simulink model "f18_SimulationModel"  (R2024a)
settings: Solver=ode1  StartTime=0.0  StopTime=200  FixedStep=0.01  RelTol=1e-3
values from neighbouring files (symbols this model uses):
  ALPHA_BREAK = [-14.0000  -10.00000   -6.00000   -2.00000    2.00000    6.00000     10.00000    14.0000    18.0000    22.0000    26.0000    30.0000    34.0000      38.0000    42.0000    46.0000    50.0000    54.0000    58.0000    62.0000      66.0000    70.0000    74.0000    78.0000    82.0000    86.0000    90.0000]*pi/180'    [f18_Aerodata.m]
  b = 37.4*0.3048    (= 11.39952)    [a1_initialize.m]
  cbar = 11.52*0.3048    (= 3.511296)    [a1_initialize.m]
  cd0 = [0.227325   0.170673    7.47685E-02    3.20977E-02    2.79305E-02  	     6.13288E-02   0.154023   0.261263   0.363863   0.486635   0.643989   0.863792  	     1.08558    1.27900    1.47638    1.61911    1.74604    1.84448    1.92402  	     1.98384    2.02834    2.06708    2.11362    2.15514    2.17363    2.16283  	     2.12822]    [f18_Aerodata.m]
  cd_de = cd_del+cd_der    [f18_Aerodata.m]
  cd_q = [ 1.48740E-16   -2.21604E-16   -8.70391E-05   -7.79330E-04   -8.31959E-04  	    -6.60720E-05    1.33279E-03    1.67685E-04    5.84481E-06   -9.59697E-17  	    -6.48262E-17   -2.05428E-16   -2.53047E-16    2.02363E-16    3.51664E-16  	     8.52635E-16    5.44982E-16   -5.45460E-16    1.14528E-15   -2.50755E-16  	     8.43503E-16   -8.45493E-16   -2.54842E-15   -7.66583E-16   -3.79368E-16  	     9.1 ...(+24 chars)    [f18_Aerodata.m]
  clift = [-1.03860  -0.880907  -0.551318  -0.216206   0.154461   0.560857  	     0.951575    1.24168    1.39786    1.53103    1.64110    1.77724    1.88652  	     1.88940    1.80975    1.68556    1.57524    1.46011    1.31884    1.17117  	     1.02151   0.858875   0.685334   0.529482   0.378268   0.229349    9.10933E-02]    [f18_Aerodata.m]
  clift_de = clift_del+clift_der    [f18_Aerodata.m]
  clift_q = [7.87143E-02    7.87143E-02    7.87144E-02    7.88452E-02    7.64891E-02  	     6.91587E-02    6.33554E-02    5.99084E-02    5.89049E-02    6.05629E-02  	     6.28755E-02    6.91587E-02    8.89245E-02    0.119991   0.147829   0.159698  	     0.131772       1.03847E-01    9.21534E-02    8.79646E-02    8.63938E-02    8.63938E-02  	     8.49975E-02    8.25541E-02    7.97615E-02    7.66200E-02    7.24 ...(+8 chars)    [f18_Aerodata.m]
  cm0 = [9.62520E-02    8.07290E-02    5.54066E-02    2.80686E-02    5.08503E-03  	    -6.61034E-03   -1.64371E-02   -1.60245E-02   -5.86329E-02   -8.42348E-02  	    -8.52663E-02  -0.105573  -0.117061  -0.110115  -0.114069  -0.118398   -1.01818E-01  	   -0.146057  -0.228343  -0.351592  -0.426319  -0.476887  -0.601749  -0.563499  	   -0.547688  -0.570013  -0.588038]    [f18_Aerodata.m]
  cm_de = cm_del+cm_der    [f18_Aerodata.m]
  cm_q = [-8.68301E-02   -8.68301E-02   -8.68301E-02   -8.65683E-02   -8.53902E-02  	    -8.08524E-02   -7.57473E-02   -7.23875E-02   -7.56600E-02   -8.29032E-02  	    -8.81828E-02   -1.02364E-01  -0.147655  -0.205556  -0.132732    1.80642E-02  	     4.31969E-02    1.80642E-02   -1.96350E-02   -6.50135E-02   -1.00967E-01  	    -9.81748E-02   -9.53822E-02   -9.25897E-02   -8.90991E-02   -8.52593E-02  	    - ...(+12 chars)    [f18_Aerodata.m]
  cn_b = [1.42071E-03    1.42071E-03    1.52521E-03    1.62971E-03    1.65089E-03  	    1.67084E-03    1.80024E-03    1.46016E-03    9.91781E-04    6.82316E-04  	    1.75902E-04   -1.09086E-03   -1.11070E-03   -1.59428E-03   -1.88776E-03  	   -1.76721E-03   -1.35917E-03   -1.52852E-03   -1.63273E-03   -1.59147E-03  	   -1.44456E-03   -1.34440E-03   -1.47796E-03   -1.60891E-03   -1.69618E-03  	    -1.72843E ...(+19 chars)    [f18_Aerodata.m]
  cn_da = [-8.69999E-06   -8.69999E-06   -8.69999E-06   -2.06625E-05   -3.45825E-05  	    -3.93675E-05   -4.78500E-05   -6.15525E-05   -7.74300E-05   -1.02660E-04  	    -1.32240E-04   -1.55512E-04   -1.72042E-04   -1.80090E-04   -1.97403E-04  	    -2.05320E-04   -2.40120E-04   -2.69352E-04   -2.87796E-04   -3.02644E-04  	    -1.09272E-04    2.45624E-12    8.35200E-05    1.59210E-04    2.21850E-04  	     2.4 ...(+24 chars)    [f18_Aerodata.m]
  cn_de = cn_del+cn_der    [f18_Aerodata.m]
  cn_dr = [-1.15493E-03   -1.15493E-03   -1.15493E-03   -1.16632E-03   -1.18177E-03  	    -1.18259E-03   -1.15656E-03   -1.08336E-03   -9.58920E-04   -8.03573E-04  	    -6.80760E-04   -6.18947E-04   -5.90480E-04   -5.80720E-04   -5.15533E-04  	    -4.17092E-04   -3.72355E-04   -3.86914E-04   -3.85538E-04   -3.51603E-04  	    -3.00387E-04   -2.75612E-04   -2.70873E-04   -3.22200E-04   -3.84710E-04  	    -4.2 ...(+24 chars)    [f18_Aerodata.m]
  cn_p = [-1.26406E-03   -1.26406E-03   -1.26406E-03   -1.23533E-03   -1.17787E-03  	    -1.12041E-03   -9.39611E-04   -6.36739E-04   -2.47236E-04    1.00356E-04  	     3.70882E-04    4.58149E-04    3.97062E-04    2.48709E-04    2.33874E-04  	     4.18879E-04    6.98132E-04    9.77384E-04   -1.04720E-03   -1.60570E-03  	    -3.24631E-04   -2.26893E-04   -1.44164E-03   -6.98132E-04   -8.81388E-14  	    -9.3 ...(+24 chars)    [f18_Aerodata.m]
  cn_r = [-3.11978E-03   -3.11978E-03   -3.11978E-03   -3.11105E-03   -3.10669E-03  	    -3.12850E-03   -3.17650E-03   -3.27686E-03   -3.46448E-03   -3.97935E-03  	    -4.62949E-03   -5.14872E-03   -5.53269E-03   -5.63741E-03   -5.53706E-03  	    -5.23162E-03   -4.53349E-03   -3.97499E-03   -2.89288E-03   -1.70606E-03  	    -6.93768E-04    4.36324E-06   -6.93769E-04   -2.64854E-03   -4.18443E-03  	    -4.8 ...(+24 chars)    [f18_Aerodata.m]
  croll_b = [-3.70196E-05   -3.70196E-05   -4.41520E-04   -8.46019E-04   -1.27065E-03  	   -1.70123E-03   -2.11290E-03   -2.77077E-03   -3.37291E-03   -3.47757E-03  	   -3.16486E-03   -2.35754E-03   -1.22554E-03   -1.14567E-03   -1.63756E-03  	   -2.22957E-03   -2.45882E-03   -2.47686E-03   -2.44493E-03   -2.51646E-03  	   -2.70976E-03   -2.90803E-03   -2.82658E-03   -2.75756E-03   -2.70552E-03  	   -2.67292E ...(+19 chars)    [f18_Aerodata.m]
  croll_da = [1.16543E-03    1.16543E-03    1.16543E-03    1.16686E-03    1.17021E-03  	    1.17426E-03    1.14013E-03    1.04034E-03    8.40294E-04    6.31892E-04  	    5.23513E-04    4.56671E-04    3.86010E-04    3.20124E-04    2.81594E-04  	    2.56481E-04    2.33946E-04    2.11792E-04    1.97660E-04    1.86966E-04  	    1.74839E-04    1.56123E-04    9.61564E-05    5.02267E-05    1.77607E-05  	   -6.65660E- ...(+18 chars)    [f18_Aerodata.m]
  croll_de = croll_del+croll_der    [f18_Aerodata.m]
  croll_dr = [2.86293E-04    2.86293E-04    2.86293E-04    2.69213E-04    2.39120E-04  	    2.18787E-04    2.10653E-04    2.07400E-04    1.80560E-04    1.24440E-04  	    6.91333E-05    3.49733E-05    1.87067E-05    4.88000E-06   -3.44528E-05  	   -8.67339E-05   -1.08661E-04   -7.83403E-05   -2.63520E-05    3.68277E-05  	    9.48021E-05    1.25253E-04    9.58432E-05    7.66811E-05    6.73115E-05  	    6.47088E- ...(+18 chars)    [f18_Aerodata.m]
  croll_p = [-7.05113E-03   -7.05113E-03   -7.05113E-03   -7.05113E-03   -7.05113E-03  	   -7.05113E-03   -6.24828E-03   -5.25344E-03   -4.62512E-03   -3.85718E-03  	   -5.38434E-03   -7.94125E-03   -8.68301E-03   -8.72665E-03   -4.88692E-03  	    3.49064E-05   -3.31613E-03   -3.73500E-03   -4.04916E-03   -4.36332E-03  	   -4.67748E-03   -4.88692E-03   -5.02655E-03   -5.16617E-03   -5.30580E-03  	   -5.41052E ...(+19 chars)    [f18_Aerodata.m]
  croll_r = [2.14676E-04    2.14676E-04    2.14676E-04    5.85558E-04    1.52804E-03  	    2.57087E-03    3.39117E-03    3.84496E-03    3.98895E-03    4.11549E-03  	    4.43401E-03    5.18886E-03    5.68192E-03    5.06669E-03    4.07360E-03  	    3.28122E-03    2.56214E-03    2.18515E-03    1.86052E-03    1.58127E-03  	    1.33692E-03    1.11352E-03    1.12748E-03    1.13097E-03    9.28515E-04  	    5.34071E- ...(+18 chars)    [f18_Aerodata.m]
  cy_b = [-1.71957E-02   -1.71957E-02   -1.77407E-02   -1.82857E-02   -1.84197E-02  	   -1.84159E-02   -1.87763E-02   -1.77142E-02   -1.55057E-02   -1.40980E-02  	   -1.28732E-02   -1.26852E-02   -1.25160E-02   -1.35594E-02   -1.40314E-02  	   -1.33128E-02   -1.19496E-02   -1.30678E-02   -1.37112E-02   -1.37528E-02  	   -1.33426E-02   -1.29076E-02   -1.33076E-02   -1.38320E-02   -1.37811E-02  	   -1.31714E ...(+19 chars)    [f18_Aerodata.m]
  cy_da = [-5.77397E-04   -5.77397E-04   -5.77397E-04   -5.46240E-04   -4.60488E-04  	   -4.06750E-04   -4.16183E-04   -3.70449E-04   -1.95515E-04    4.51627E-05  	    2.63830E-04    4.73923E-04    6.38852E-04    7.09741E-04    6.50343E-04  	    1.99345E-04   -1.00616E-04   -1.48179E-04   -1.74477E-04   -1.95743E-04  	   -2.18725E-04   -2.40677E-04   -2.78179E-04   -3.06420E-04   -3.28602E-04  	   -3.47581E ...(+19 chars)    [f18_Aerodata.m]
  cy_de = cy_del+cy_der    [f18_Aerodata.m]
  cy_dr = [3.46480E-03    3.46480E-03    3.46480E-03    3.52987E-03    3.66813E-03  	    3.73320E-03    3.66813E-03    3.46480E-03    3.08253E-03    2.57827E-03  	    2.11467E-03    1.79747E-03    1.59413E-03    1.47213E-03    1.50955E-03  	    1.59771E-03    1.48189E-03    1.25806E-03    1.04497E-03    9.72747E-04  	    1.04790E-03    1.15331E-03    1.10125E-03    1.01504E-03    1.04757E-03  	    1.15266E- ...(+18 chars)    [f18_Aerodata.m]
  cy_p = [-1.06465E-03   -1.06465E-03   -1.06465E-03   -8.63938E-04   -2.09440E-04  	    4.14516E-04    5.80322E-04    5.32325E-04    4.53786E-04    2.22529E-04  	   -1.74533E-04   -5.49779E-04   -9.42478E-04   -1.35699E-03   -2.60752E-03  	   -4.39823E-03   -5.23599E-03   -3.00197E-03   -1.65806E-03   -7.85399E-04  	   -2.96706E-04   -4.36332E-04   -9.25024E-04   -9.94838E-04   -9.25024E-04  	   -9.77384E ...(+19 chars)    [f18_Aerodata.m]
  cy_r = [2.69653E-03    2.69653E-03    2.69653E-03    2.89725E-03    3.36412E-03  	    3.94444E-03    4.45932E-03    3.82227E-03    1.22609E-03   -1.61443E-03  	   -3.46448E-03   -4.66876E-03   -5.36689E-03   -5.67232E-03   -3.89208E-03  	    3.49069E-05    5.06146E-03    5.06145E-03    4.11898E-03    2.79253E-03  	    1.60570E-03    1.04720E-03    8.37758E-04    6.28319E-04    4.88692E-04  	    4.18879E- ...(+18 chars)    [f18_Aerodata.m]
  g = 9.80665    [a1_initialize.m]
  InertiaTensor = [Ixx 0 -Ixz; 0 Iyy 0; -Ixz 0 Izz]    [a1_initialize.m]
  init_eulers = x0(7:9)    [a1_initialize.m]
  init_inertial = x0(10:12)    [a1_initialize.m]
  init_omega_b = x0(1:3)    [a1_initialize.m]
  init_Vb = x0(4:6)    [a1_initialize.m]
  mass = 36100/2.2046    (= 16374.852581)    [a1_initialize.m]
  max_thrust = 32000*g/2.2046    (= 142344.5523)    [a1_initialize.m]
  rho_sl = 1.225    [a1_initialize.m]
  S = 400.0*0.3048*0.3048    (= 37.161216)    [a1_initialize.m]
undefined symbols (not defined in the file or in its folder): Earth, WGS84
libraries: aerolibfltsims x2, matrix_library x2, aerolibtransform2 x1, Rotation_Matrices_All x1
(part 1 of 2)
settings Model: Creator=ragup  LastModifiedBy=ragup
settings DataIOCC: ExternalInput=getinputstruct(opreport)  InitialState=getstatestruct(opreport)  LoadExternalInput=on  LoadInitialState=on  SaveOutput=off  SignalLogging=off  DSMLogging=off  SaveTime=off  ReturnWorkspaceOutputs=off

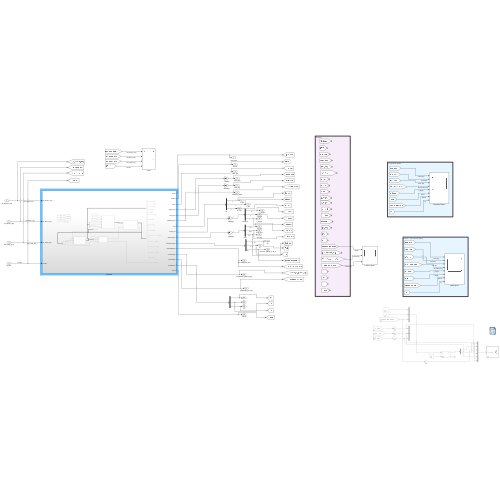
[thumbnail: Simulink's stored preview of the top-level diagram]
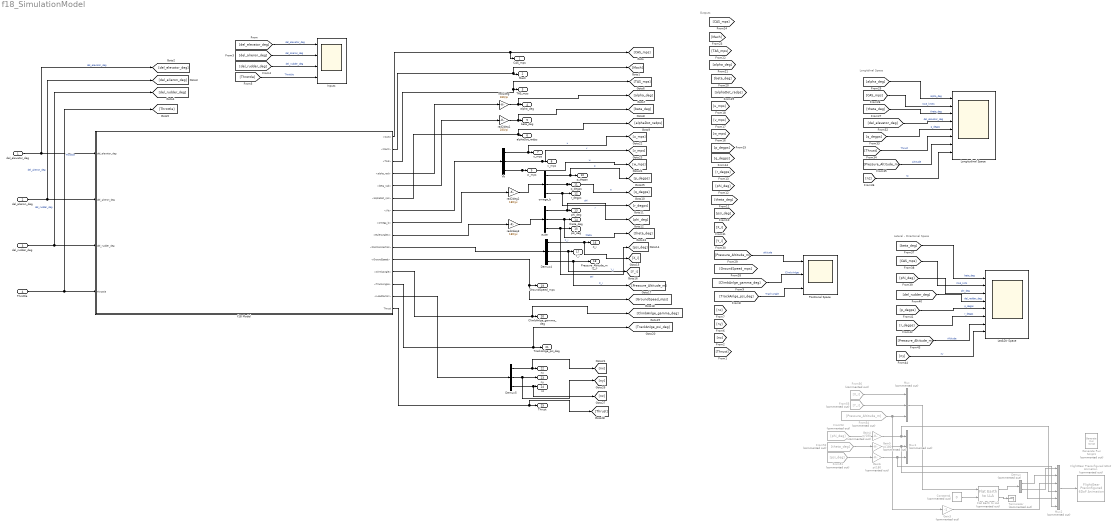
== system f18_SimulationModel ==
  note: Outputs
  note: Longitdinal Space
  note: Lateral - Directional Space
  del_elevator_deg : Inport
  del_alieron_deg : Inport  Port=2
  del_rudder_deg : Inport  Port=3
  Throttle : Inport  Port=4
  Constant4 : Constant  Commented=on  Value=0
  Demux : Demux  Commented=on  Outputs=2
  Demux4 : Demux  Outputs=3
  Demux5 : Demux  Outputs=3
  Flat Earth to LLA : aerolibtransform2/Flat Earth to LLA  Commented=on  units=Metric (MKS)  ptype=Earth (WGS84)  F=1/298.257223563  R=6378137  refPosPort=off  LL0=[63 -22]  psi=0
  FlightGear Preconfigured 6DoF Animation : aerolibfltsims/FlightGear Preconfigured 6DoF Animation  Commented=on  xFlightGearVersion=v2019.1  DestinationIpAddress=127.0.0.1  DestinationPort=5502  SampleTime=0.01  packetVersion=24
  From51 : From  Commented=on  GotoTag=psi_deg
  From52 : From  Commented=on  GotoTag=theta_deg
  From53 : From  Commented=on  GotoTag=phi_deg
  From54 : From  Commented=on  GotoTag=Pressure_Altitude_m
  From55 : From  Commented=on  GotoTag=Y_i
  From56 : From  Commented=on  GotoTag=X_i
  Gain3 : Gain  Commented=on  Gain=-1
  Gain4 : Gain  Commented=on  Gain=pi/180
  Gain5 : Gain  Commented=on  Gain=pi/180
  Gain6 : Gain  Commented=on  Gain=pi/180
  Generate Run Script1 : aerolibfltsims/Generate Run Script  Commented=on  Architecture=Win64  dataFlow=Send  GeometryModelName=c172p  AirportId=BIKF  RunwayId=10  InitialAltitude=2000  InitialHeading=0  OffsetDistance=4.7  OffsetAzimuth=0  InstallScenery=off  DisableShaders=off  OriginAddress=127.0.0.1  DestinationPort=5502  OriginPort=5505  LocalAddress=127.0.0.1  OutputFileName=runfg_f18.bat  FlightGearBaseDirectory=C:\Program Files\FlightGear
  Inputs : Scope  NumInputPorts=4
  Lat&Dir Space : Scope  NumInputPorts=8
  Longitudinal Space : Scope  NumInputPorts=8
  Mux : Mux  Commented=on  Inputs=3
  Mux1 : Mux  Commented=on  Inputs=3
  Mux2 : Mux  Commented=on  Inputs=6
  Positional Space : Scope  NumInputPorts=3
  Terminator : Terminator  Commented=on
  Vb : Demux  Outputs=3
  euler : Demux  Outputs=3
  f18 Model : Subsystem
  omega_b : Demux  Outputs=3
  rad2deg{,1..3} (4 alike) : Gain  Gain=180/pi
  CAS_mps : Outport
  Mach : Outport  Port=2
  TAS_mps : Outport  Port=3
  alpha_deg : Outport  Port=4
  beta_deg : Outport  Port=5
  alphaDot_radps : Outport  Port=6
  u_mps : Outport  Port=7
  v_mps : Outport  Port=8
  w_mps : Outport  Port=9
  p_degps : Outport  Port=10
  q_degps : Outport  Port=11
  r_degps : Outport  Port=12
  phi_deg : Outport  Port=13
  theta_deg : Outport  Port=14
  psi_deg : Outport  Port=15
  X_i : Outport  Port=16
  Y_i : Outport  Port=17
  Pressure_Altitude_m (Z_i) : Outport  Port=18
  GroundSpeed_mps : Outport  Port=19
  ClimbAnlge_gamma_deg : Outport  Port=20
  TrackAnlge_psi_deg : Outport  Port=21
  nx : Outport  Port=22
  ny : Outport  Port=23
  nz : Outport  Port=24
  Thrust : Outport  Port=25
  wires:
  rad2deg/1 -> [alpha_deg], alpha_deg/1
  rad2deg1/1 -> [beta_deg], beta_deg/1
  Vb/1 -> [u_mps], u_mps/1  "u"
  Vb/2 -> [v_mps], v_mps/1  "v"
  Vb/3 -> [w_mps], w_mps/1  "w"
  omega_b/3 -> [r_degps], r_degps/1  "r"
  omega_b/2 -> [q_degps], q_degps/1  "q"
  omega_b/1 -> [p_degps], p_degps/1  "p"
  rad2deg2/1 -> omega_b/1
  rad2deg3/1 -> euler/1
  euler/1 -> [phi_deg], phi_deg/1  "phi"
  euler/2 -> [theta_deg], theta_deg/1  "theta"
  euler/3 -> [psi_deg], psi_deg/1  "psi"
  Demux4/3 -> Pressure_Altitude_m (Z_i)/1, [Pressure_Altitude_m]  "Z_i"
  Demux4/2 -> [Y_i], Y_i/1  "Y_i"
  Demux4/1 -> [X_i], X_i/1  "X_i"
  Demux5/3 -> [nz], nz/1
  Demux5/1 -> [nx], nx/1
  Demux5/2 -> ny/1, [ny]
  [beta_deg] -> Lat&Dir Space/1  "beta_deg"
  [q_degps] -> Longitudinal Space/5  "q_degps"
  [nz] -> Longitudinal Space/8  "nz"
  [Pressure_Altitude_m] -> Longitudinal Space/7  "Altitude"
  [theta_deg] -> Longitudinal Space/3  "theta_deg"
  [alpha_deg] -> Longitudinal Space/1  "alpha_deg"
  [del_rudder_deg] -> Lat&Dir Space/4  "del_redder_deg"
  [Pressure_Altitude_m] -> Lat&Dir Space/7  "Altitude"
  [ny] -> Lat&Dir Space/8  "ny"
  [r_degps] -> Lat&Dir Space/6  "r_degps"
  [CAS_mps] -> Lat&Dir Space/2  "CAS_knts"
  [CAS_mps] -> Longitudinal Space/2  "CAS_knots"
  [del_elevator_deg] -> Longitudinal Space/4  "del_elevator_deg"
  [p_degps] -> Lat&Dir Space/5  "p_degps"
  [Thrust] -> Longitudinal Space/6  "Thrust"
  [phi_deg] -> Lat&Dir Space/3  "phi_deg"
  f18 Model/15(Thrust) -> [Thrust], Thrust/1
  f18 Model/12(<ClimbAngle>) -> [ClimbAnlge_gamma_deg], ClimbAnlge_gamma_deg/1
  f18 Model/13(<TrackAngle>) -> [TrackAnlge_psi_deg], TrackAnlge_psi_deg/1
  f18 Model/11(<GroundSpeed>) -> GroundSpeed_mps/1, [GroundSpeed_mps]
  f18 Model/2(<Mach>) -> [Mach], Mach/1
  f18 Model/3(<TAS>) -> [TAS_mps], TAS_mps/1
  f18 Model/1(<CAS>) -> CAS_mps/1, [CAS_mps]
  f18 Model/6(<alphaDot_rps>) -> [alphaDot_radps], alphaDot_radps/1
  f18 Model/4(<alpha_rad>) -> rad2deg/1
  f18 Model/5(<beta_rad>) -> rad2deg1/1
  f18 Model/7(<Vb>) -> Vb/1
  f18 Model/8(<omega_b>) -> rad2deg2/1
  f18 Model/9(<EulerAngles>) -> rad2deg3/1
  f18 Model/10(<PositionInertial>) -> Demux4/1
  f18 Model/14(<LoadFactor>) -> Demux5/1
  Flat Earth to LLA/1 -> Demux/1
  Gain5/1 -> Mux2/5, Mux1/2
  Gain6/1 -> Mux1/3, Mux2/6
  Gain3/1 -> Mux2/3
  Gain4/1 -> Mux2/4, Mux1/1
  From56/1 -> Mux/1
  Mux2/1 -> FlightGear Preconfigured 6DoF Animation/1
  Flat Earth to LLA/2 -> Terminator/1
  Demux/2 -> Mux2/1
  From52/1 -> Gain5/1
  Constant4/1 -> Flat Earth to LLA/2
  Mux/1 -> Flat Earth to LLA/1
  From51/1 -> Gain6/1
  From53/1 -> Gain4/1
  Demux/1 -> Mux2/2
  From54/1 -> Gain3/1, Mux/3
  From55/1 -> Mux/2
  [del_elevator_deg] -> Inputs/1  "del_elevator_deg"
  [del_alieron_deg] -> Inputs/2  "del_alieron_deg"
  [del_rudder_deg] -> Inputs/3  "del_rudder_deg"
  [Throttle] -> Inputs/4  "Throttle"
  del_elevator_deg/1 -> [del_elevator_deg], f18 Model/1(del_elevator_deg)  "del_elevator_deg"
  del_alieron_deg/1 -> [del_alieron_deg], f18 Model/2(del_alieron_deg)  "del_alieron_deg"
  del_rudder_deg/1 -> [del_rudder_deg], f18 Model/3(del_rudder_deg)  "del_rudder_deg"
  Throttle/1 -> [Throttle], f18 Model/4(Throttle)  "Throttle"
  [ClimbAnlge_gamma_deg] -> Positional Space/2  "Climb Anlge"
  [TrackAnlge_psi_deg] -> Positional Space/3  "Trach Angle"
  [Pressure_Altitude_m] -> Positional Space/1  "altitude"

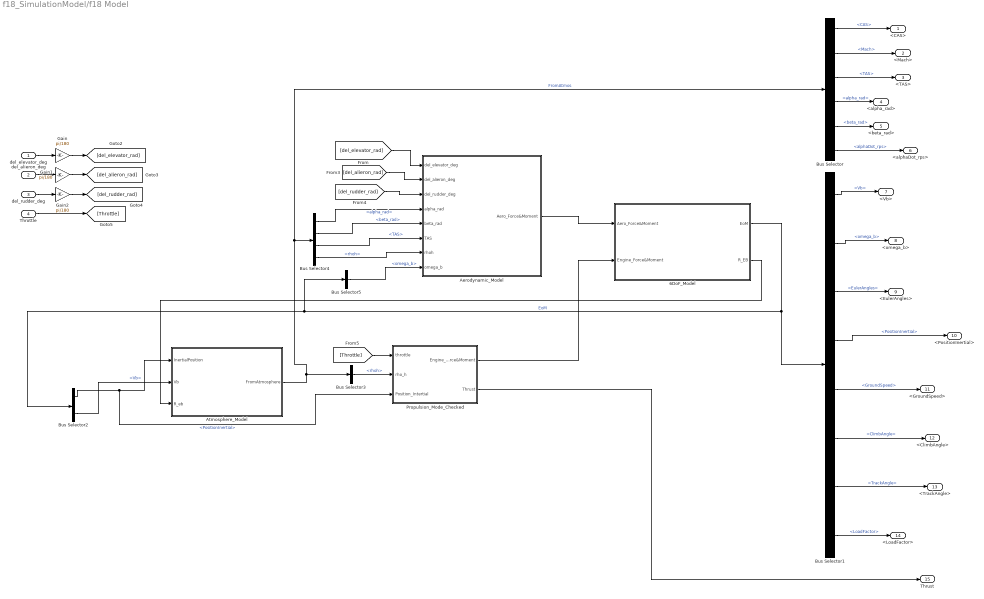
== system f18_SimulationModel/f18 Model ==
  del_elevator_deg : Inport
  del_alieron_deg : Inport  Port=2
  del_rudder_deg : Inport  Port=3
  Throttle : Inport  Port=4
  6DoF_Model : Subsystem
  Aerodynamic_Model : Subsystem
  Atmosphere_Model : Subsystem
  Bus Selector : BusSelector  OutputSignals=CAS,Mach,TAS,alpha_rad,beta_rad,alphaDot_rps
  Bus Selector1 : BusSelector  OutputSignals=Vb,omega_b,EulerAngles,PositionInertial,GroundSpeed,ClimbAngle,TrackAngle,LoadFactor
  Bus Selector2 : BusSelector  OutputSignals=PositionInertial,Vb
  Bus Selector3 : BusSelector  OutputSignals=rhoh
  Bus Selector4 : BusSelector  OutputSignals=alpha_rad,beta_rad,TAS,rhoh
  Bus Selector5 : BusSelector  OutputSignals=omega_b
  Gain : Gain  Gain=pi/180
  Gain1 : Gain  Gain=pi/180
  Gain2 : Gain  Gain=pi/180
  Propulsion_Mode_Checked : Subsystem
  <CAS> : Outport
  <Mach> : Outport  Port=2
  <TAS> : Outport  Port=3
  <alpha_rad> : Outport  Port=4
  <beta_rad> : Outport  Port=5
  <alphaDot_rps> : Outport  Port=6
  <Vb> : Outport  Port=7
  <omega_b> : Outport  Port=8
  <EulerAngles> : Outport  Port=9
  <PositionInertial> : Outport  Port=10
  <GroundSpeed> : Outport  Port=11
  <ClimbAngle> : Outport  Port=12
  <TrackAngle> : Outport  Port=13
  <LoadFactor> : Outport  Port=14
  Thrust : Outport  Port=15
  wires:
  Atmosphere_Model/1(FromAtmosphere) -> Bus Selector/1, Bus Selector4/1, Bus Selector3/1  "FromAtmos"
  Bus Selector4/1 -> Aerodynamic_Model/4(alpha_rad)  "<alpha_rad>"
  Propulsion_Mode_Checked/1(Engine_Force&Moment) -> 6DoF_Model/2(Engine_Force&Moment)
  Bus Selector2/2 -> Atmosphere_Model/2(Vb)  "<Vb>"
  Aerodynamic_Model/1(Aero_Force&Moment) -> 6DoF_Model/1(Aero_Force&Moment)
  Propulsion_Mode_Checked/2(Thrust) -> Thrust/1
  [del_elevator_rad] -> Aerodynamic_Model/1(del_elevator_deg)
  Bus Selector1/7 -> <TrackAngle>/1  "<TrackAngle>"
  del_elevator_deg/1 -> Gain/1
  Bus Selector/2 -> <Mach>/1  "<Mach>"
  [del_rudder_rad] -> Aerodynamic_Model/3(del_rudder_deg)
  Bus Selector/6 -> <alphaDot_rps>/1  "<alphaDot_rps>"
  Bus Selector3/1 -> Propulsion_Mode_Checked/2(rho_h)  "<rhoh>"
  del_alieron_deg/1 -> Gain1/1
  Bus Selector4/3 -> Aerodynamic_Model/6(TAS)  "<TAS>"
  Bus Selector4/4 -> Aerodynamic_Model/7(rhoh)  "<rhoh>"
  Bus Selector4/2 -> Aerodynamic_Model/5(beta_rad)  "<beta_rad>"
  Bus Selector2/1 -> Propulsion_Mode_Checked/3(Position_Intertial), Atmosphere_Model/1(InertialPosition)  "<PositionInertial>"
  6DoF_Model/1(EoM) -> Bus Selector5/1, Bus Selector2/1, Bus Selector1/1  "EoM"
  [del_alieron_rad] -> Aerodynamic_Model/2(del_alieron_deg)
  Bus Selector5/1 -> Aerodynamic_Model/8(omega_b)  "<omega_b>"
  Bus Selector1/8 -> <LoadFactor>/1  "<LoadFactor>"
  6DoF_Model/2(R_EB) -> Atmosphere_Model/3(R_eb)
  Bus Selector1/2 -> <omega_b>/1  "<omega_b>"
  [Throttle] -> Propulsion_Mode_Checked/1(throttle)
  del_rudder_deg/1 -> Gain2/1
  Bus Selector1/5 -> <GroundSpeed>/1  "<GroundSpeed>"
  Bus Selector/4 -> <alpha_rad>/1  "<alpha_rad>"
  Throttle/1 -> [Throttle]
  Bus Selector1/1 -> <Vb>/1  "<Vb>"
  Bus Selector1/3 -> <EulerAngles>/1  "<EulerAngles>"
  Bus Selector1/6 -> <ClimbAngle>/1  "<ClimbAngle>"
  Bus Selector1/4 -> <PositionInertial>/1  "<PositionInertial>"
  Bus Selector/1 -> <CAS>/1  "<CAS>"
  Bus Selector/3 -> <TAS>/1  "<TAS>"
  Bus Selector/5 -> <beta_rad>/1  "<beta_rad>"
  Gain/1 -> [del_elevator_rad]
  Gain1/1 -> [del_alieron_rad]
  Gain2/1 -> [del_rudder_rad]

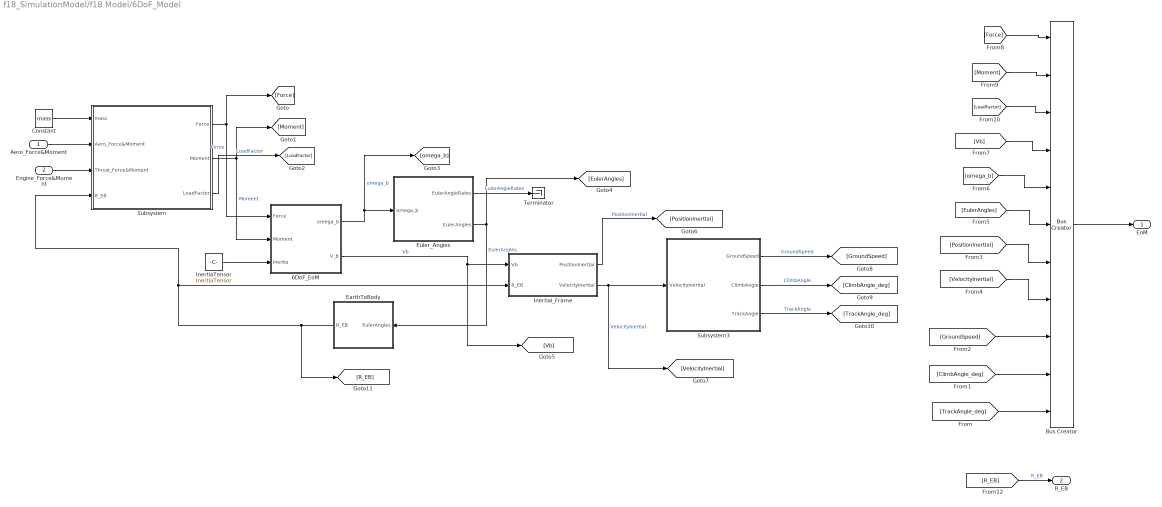
== system f18_SimulationModel/f18 Model/6DoF_Model ==
  Aero_Force&Moment : Inport
  Engine_Force&Moment : Inport  Port=2
  6DoF_EoM : Subsystem
  Bus Creator : BusCreator  Inputs=11
  Constant : Constant  Value=mass
  EarthToBody : Subsystem
  Euler_Angles : Subsystem
  InertiaTensor : Constant  Value=InertiaTensor  VectorParams1D=off
  Inertial_Frame : Subsystem
  Subsystem : Subsystem
  Subsystem3 : Subsystem
  Terminator : Terminator
  EoM : Outport
  R_EB : Outport  Port=2
  wires:
  [ClimbAngle_deg] -> Bus Creator/10
  [LoadFactor] -> Bus Creator/3
  [Moment] -> Bus Creator/2
  Bus Creator/1 -> EoM/1
  Subsystem/3(LoadFactor) -> [LoadFactor]  "LoadFactor"
  [PositionInertial] -> Bus Creator/7
  Inertial_Frame/1(PositionInertial) -> [PositionInertial]  "PositionInertial"
  [omega_b] -> Bus Creator/5
  EarthToBody/1(R_EB) -> [R_EB], Inertial_Frame/2(R_EB), Subsystem/4(R_EB)
  Euler_Angles/1(EulerAngleRates) -> Terminator/1  "EulerAngleRates"
  Subsystem3/1(GroundSpeed) -> [GroundSpeed]  "GroundSpeed"
  Aero_Force&Moment/1 -> Subsystem/2(Aero_Force&Moment)
  Subsystem3/2(ClimbAngle) -> [ClimbAngle_deg]  "ClimbAngle"
  [EulerAngles] -> Bus Creator/6
  [VelocityInertial] -> Bus Creator/8
  [GroundSpeed] -> Bus Creator/9
  6DoF_EoM/2(V_b) -> Inertial_Frame/1(Vb), [Vb]  "Vb"
  Engine_Force&Moment/1 -> Subsystem/3(Thrust_Force&Moment)
  [Force] -> Bus Creator/1
  Constant/1 -> Subsystem/1(mass)
  Inertial_Frame/2(VelocityInertial) -> Subsystem3/1(VelocityInertial), [VelocityInertial]  "VelocityInertial"
  [TrackAngle_deg] -> Bus Creator/11
  [Vb] -> Bus Creator/4
  6DoF_EoM/1(omega_b) -> [omega_b], Euler_Angles/1(omega_b)  "omega_b"
  Euler_Angles/2(EulerAngles) -> [EulerAngles], EarthToBody/1(EulerAngles)  "EulerAngles"
  Subsystem/2(Moment) -> [Moment], 6DoF_EoM/2(Moment)  "Moment"
  Subsystem3/3(TrackAngle) -> [TrackAngle_deg]  "TrackAngle"
  Subsystem/1(Force) -> [Force], 6DoF_EoM/1(Force)  "Force"
  [R_EB] -> R_EB/1  "R_EB"
  InertiaTensor/1 -> 6DoF_EoM/3(Inertia)

== system f18_SimulationModel/f18 Model/Aerodynamic_Model ==
  del_elevator_deg : Inport
  del_alieron_deg : Inport  Port=2
  del_rudder_deg : Inport  Port=3
  alpha_rad : Inport  Port=4
  beta_rad : Inport  Port=5
  TAS : Inport  Port=6
  rhoh : Inport  Port=7
  omega_b : Inport  Port=8
  Absolute Force&Moment : Subsystem
  Bus Creator1 : BusCreator  Inputs=6
  Co-efficent Calculation in body FoR : Subsystem
  Demux : Demux  Outputs=3
  Demux4 : Demux  Outputs=2
  Demux5 : Demux  Outputs=3
  Demux6 : Demux  Outputs=3
  Stability FoR to Body FoR : Subsystem
  Aero_Force&Moment : Outport
  wires:
  Demux/1 -> Co-efficent Calculation in body FoR/3(p)  "p"
  omega_b/1 -> Demux/1
  [TAS] -> Co-efficent Calculation in body FoR/9(TAS)
  TAS/1 -> [TAS]
  rhoh/1 -> [rhoh]
  Demux/2 -> Co-efficent Calculation in body FoR/4(q)  "q"
  alpha_rad/1 -> Stability FoR to Body FoR/1(alpha_rad), Co-efficent Calculation in body FoR/1(alpha_rad)
  del_alieron_deg/1 -> Co-efficent Calculation in body FoR/7(del_alieron_deg)
  Demux/3 -> Co-efficent Calculation in body FoR/5(r)  "r"
  del_elevator_deg/1 -> Co-efficent Calculation in body FoR/6(del_elevator_deg)
  beta_rad/1 -> Co-efficent Calculation in body FoR/2(beta_rad)
  del_rudder_deg/1 -> Co-efficent Calculation in body FoR/8(del_rudder_deg)
  Bus Creator1/1 -> Aero_Force&Moment/1
  Demux4/1 -> Demux5/1  "AeroForce_bFoR"
  Demux5/1 -> Bus Creator1/1  "X_Aero"
  Demux6/1 -> Bus Creator1/4  "L_Aero"
  Demux6/2 -> Bus Creator1/5  "M_aero"
  Demux5/2 -> Bus Creator1/2  "Y_Aero"
  Demux4/2 -> Demux6/1  "AeroMoment_b_AC"
  [rhoh] -> Absolute Force&Moment/1(rhoh)
  Stability FoR to Body FoR/2(AeroMoment_Coefficients_b_AC) -> Absolute Force&Moment/4(CM)  "AeroMoment_Coefficients_b_AC"
  Demux5/3 -> Bus Creator1/3  "Z_Aero"
  Stability FoR to Body FoR/1(AeroForce_Coefficients_bFoR) -> Absolute Force&Moment/3(CF)  "AeroForce_Coefficients_bFoR"
  Absolute Force&Moment/1(Aero_Force&Moment_ac) -> Demux4/1  "Aero_Force&Moment_ac"
  Demux6/3 -> Bus Creator1/6  "N_aero"
  [TAS] -> Absolute Force&Moment/2(TAS)
  Co-efficent Calculation in body FoR/1(CL) -> Stability FoR to Body FoR/2(CL)  "CL"
  Co-efficent Calculation in body FoR/2(CD) -> Stability FoR to Body FoR/3(CD)  "CD"
  Co-efficent Calculation in body FoR/3(CY) -> Stability FoR to Body FoR/4(CY)  "CY"
  Co-efficent Calculation in body FoR/4(Cl) -> Stability FoR to Body FoR/5(Cl)  "Cl"
  Co-efficent Calculation in body FoR/5(Cm) -> Stability FoR to Body FoR/6(Cm)  "Cm"
  Co-efficent Calculation in body FoR/6(Cn) -> Stability FoR to Body FoR/7(Cn)  "Cn"

== system f18_SimulationModel/f18 Model/Atmosphere_Model ==
  InertialPosition : Inport
  Vb : Inport  Port=2
  R_eb : Inport  Port=3
  Bus Creator : BusCreator  Inputs=10
  Constant : Constant  Value=0
  Demux : Demux  Outputs=3
  EoM&Wind --> TAS : Subsystem
  Gain : Gain  Gain=-1
  ISA_upto20km : Subsystem
      mask Display: image('ISA_Temperature.png', [3,3,3,3,100,100]);
  TAS2CAS : Subsystem
      mask Display: image('TAS2CAS.png', [3,3,3,3,100,100]);
  Terminator : Terminator
  Terminator1 : Terminator
  FromAtmosphere : Outport
  wires:
  Demux/3 -> Gain/1
  Demux/2 -> Terminator1/1
  Demux/1 -> Terminator/1
  InertialPosition/1 -> Demux/1
  ISA_upto20km/4(ah) -> TAS2CAS/2(ah), Bus Creator/1  "ah"
  Gain/1 -> ISA_upto20km/1(h)
  Bus Creator/1 -> FromAtmosphere/1
  EoM&Wind --> TAS/4(aplhaDot_rps) -> Bus Creator/10  "alphaDot_rps"
  ISA_upto20km/2(Ph) -> Bus Creator/3, TAS2CAS/1(Ph)  "Ph"
  ISA_upto20km/1(Th) -> Bus Creator/2  "Th"
  TAS2CAS/1(Mach) -> Bus Creator/5  "Mach"
  EoM&Wind --> TAS/1(TAS) -> Bus Creator/7, TAS2CAS/3(TAS)  "TAS"
  EoM&Wind --> TAS/2(alpha_rad) -> Bus Creator/8  "alpha_rad"
  EoM&Wind --> TAS/3(beta_rad) -> Bus Creator/9  "beta_rad"
  TAS2CAS/2(CAS) -> Bus Creator/6  "CAS"
  ISA_upto20km/3(rhoh) -> Bus Creator/4  "rhoh"
  Constant/1 -> EoM&Wind --> TAS/1(Wind_InertialX), EoM&Wind --> TAS/3(Wind_InertialZ), EoM&Wind --> TAS/2(Wind_InertialY)
  R_eb/1 -> EoM&Wind --> TAS/4(R_EB)
  Vb/1 -> EoM&Wind --> TAS/5(Vb)

== system f18_SimulationModel/f18 Model/Propulsion_Mode_Checked ==
  throttle : Inport
  rho_h : Inport  Port=2
  Position_Intertial : Inport  Port=3
  Constant : Constant  Value=0
  Demux : Demux  Outputs=3
  Gain : Gain  Gain=-1
  Mux : Mux  Inputs=6
  Mux2 : Mux  Inputs=3
  Stengel Model : Fcn  Expr=((u(2)/rho_sl)^0.7)*max_thrust*(1-exp((u(3)-17000)/2000))*u(1);
  Terminator : Terminator
  Terminator1 : Terminator
  Engine_Force&Moment : Outport
  Thrust : Outport  Port=2
  wires:
  Stengel Model/1 -> Thrust/1, Mux/1
  Constant/1 -> Mux/2, Mux/3, Mux/6, Mux/5, Mux/4
  Mux/1 -> Engine_Force&Moment/1
  Mux2/1 -> Stengel Model/1
  throttle/1 -> Mux2/1
  rho_h/1 -> Mux2/2
  Gain/1 -> Mux2/3
  Demux/3 -> Gain/1
  Demux/1 -> Terminator/1
  Demux/2 -> Terminator1/1
  Position_Intertial/1 -> Demux/1

== system f18_SimulationModel/f18 Model/6DoF_Model/6DoF_EoM ==
  Force : Inport
  Moment : Inport  Port=2
  Inertia : Inport  Port=3
  Rotational_EoM : Subsystem
  Translational_EoM : Subsystem
  omega_b : Outport
  V_b : Outport  Port=2
  wires:
  Moment/1 -> Rotational_EoM/1(Moment)
  Translational_EoM/1(V_b) -> V_b/1
  Force/1 -> Translational_EoM/1(Force)
  Inertia/1 -> Rotational_EoM/2(Inertia)
  Rotational_EoM/1(omega_b) -> omega_b/1, Translational_EoM/2(omega)

== system f18_SimulationModel/f18 Model/6DoF_Model/EarthToBody ==
  EulerAngles : Inport
  Demux : Demux  Outputs=3
  Product1 : Product  Multiplication=Matrix(*)
  Product2 : Product  Multiplication=Matrix(*)
  Subsystem2 : Subsystem
  Subsystem3 : Subsystem
  Subsystem4 : Subsystem
  R_EB : Outport
  wires:
  Demux/3 -> Subsystem2/1(psi)  "psi"
  Demux/2 -> Subsystem4/1(theta)  "theta"
  EulerAngles/1 -> Demux/1  "EulerAngles"
  Demux/1 -> Subsystem3/1(phi)  "phi"
  Product2/1 -> R_EB/1
  Product1/1 -> Product2/1
  Subsystem2/1(R_psi) -> Product2/2
  Subsystem4/1(R_theta) -> Product1/2
  Subsystem3/1(R_phi) -> Product1/1

== system f18_SimulationModel/f18 Model/6DoF_Model/Euler_Angles ==
  omega_b : Inport
  Abs : Abs  SaturateOnIntegerOverflow=off
  Constant : Constant  Value=0.001
  Demux : Demux  Outputs=3
  Demux1 : Demux  Outputs=3
  Fcn : Fcn  Expr=u(1) + (u(2)*u(4)*u(5)/u(8)) + (u(3)*u(7)*u(5)/u(8))
  Fcn1 : Fcn  Expr=(u(2)*u(7)) - (u(3)*u(4))
  Fcn2 : Fcn  Expr=((u(2)*u(4)) + (u(3)*u(7))) / u(8)
  Mux{,1..3} (4 alike) : Mux  Inputs=3
  Product : Product
  Relay : Relay  OnSwitchValue=0.001  OffSwitchValue=0  OnOutputValue=0  OffOutputValue=1
  Sign : Signum
  Switch : Switch  Criteria=u2 > Threshold  Threshold=0.5  SaturateOnIntegerOverflow=off  InputSameDT=off
  Trigonometric Function : Trigonometry  Operator=sincos
  phi_dot : Integrator  InitialCondition=init_eulers(1)  ContinuousStateAttributes='phi_dot'
  psi_dot : Integrator  InitialCondition=init_eulers(3)  ContinuousStateAttributes='psi_dot'
  theta_dot : Integrator  InitialCondition=init_eulers(2)  ContinuousStateAttributes='theta_dot'
  EulerAngleRates : Outport
  EulerAngles : Outport  Port=2
  wires:
  Mux3/1 -> EulerAngles/1, Trigonometric Function/1  "EulerAngles"
  phi_dot/1 -> Mux3/1  "phi"
  Demux1/3 -> psi_dot/1  "psi_dot"
  Mux2/1 -> Demux1/1, EulerAngleRates/1
  Demux1/2 -> theta_dot/1  "theta_dot"
  theta_dot/1 -> Mux3/2  "theta"
  Demux1/1 -> phi_dot/1  "phi_dot"
  psi_dot/1 -> Mux3/3  "psi"
  Fcn2/1 -> Mux2/3  "psi_dot"
  Mux/1 -> Mux1/3
  Constant/1 -> Product/1
  Demux/1 -> Mux/1  "cos(phi)"
  Fcn1/1 -> Mux2/2  "theta_dot"
  Demux/3 -> Mux/3  "cos(psi)"
  Switch/1 -> Mux/2
  Mux1/1 -> Fcn1/1, Fcn2/1, Fcn/1
  Sign/1 -> Product/2
  Abs/1 -> Relay/1
  Fcn/1 -> Mux2/1  "phi_dot"
  Relay/1 -> Switch/2
  Product/1 -> Switch/1
  omega_b/1 -> Mux1/1
  Trigonometric Function/2 -> Demux/1
  Trigonometric Function/1 -> Mux1/2
  Demux/2 -> Abs/1, Switch/3, Sign/1  "cos(theta)"

== system f18_SimulationModel/f18 Model/6DoF_Model/Inertial_Frame ==
  Vb : Inport
  R_EB : Inport  Port=2
  Demux : Demux  Outputs=3
  Demux1 : Demux  Outputs=3
  Gain : Gain  Gain=-1
  Matrix Multiply : Product  Multiplication=Matrix(*)
  Mux : Mux  Inputs=3
  Mux1 : Mux  Inputs=3
  Transpose : Math  Operator=transpose
  Xi_dot : Integrator  InitialCondition=init_inertial(1)  ContinuousStateAttributes='Xi_dot'
  Yi_dot : Integrator  InitialCondition=init_inertial(2)  ContinuousStateAttributes='Yi_dot'
  Zi_dot : Integrator  InitialCondition=init_inertial(3)  ContinuousStateAttributes='Zi_dot'
  PositionInertial : Outport
  VelocityInertial : Outport  Port=2
  wires:
  R_EB/1 -> Transpose/1
  Transpose/1 -> Matrix Multiply/1  "R_BE"
  Vb/1 -> Matrix Multiply/2
  Demux/3 -> Zi_dot/1  "Zi_dot"
  Mux/1 -> PositionInertial/1
  Xi_dot/1 -> Mux/1  "Xi"
  Demux/1 -> Xi_dot/1  "Xi_dot"
  Demux/2 -> Yi_dot/1  "Yi_dot"
  Yi_dot/1 -> Mux/2  "Yi"
  Zi_dot/1 -> Mux/3  "Zi"
  Mux1/1 -> VelocityInertial/1, Demux/1
  Matrix Multiply/1 -> Demux1/1
  Demux1/1 -> Mux1/1  "Xi_dot"
  Demux1/2 -> Mux1/2  "Yi_dot"
  Demux1/3 -> Gain/1
  Gain/1 -> Mux1/3  "Zi_dot"

== system f18_SimulationModel/f18 Model/6DoF_Model/Subsystem ==
  mass : Inport
  Aero_Force&Moment : Inport  Port=2
  Thrust_Force&Moment : Inport  Port=3
  R_EB : Inport  Port=4
  Add : Sum
  Constant : Constant  Value=0
  Demux : Demux  Outputs=2
  Demux1 : Demux  Outputs=3
  Divide : Product  Inputs=*/  Multiplication=Matrix(*)
  Gain : Gain  Gain=g
  Gain1 : Gain  Gain=-1
  Mux : Mux  Inputs=3
  Mux1 : Mux  Inputs=3
  Product : Product  Multiplication=Matrix(*)
  Sum : Sum  Inputs=|++
  Force : Outport
  Moment : Outport  Port=2
  LoadFactor : Outport  Port=3
  wires:
  Demux1/3 -> Gain1/1
  Mux1/1 -> LoadFactor/1
  Mux/1 -> Product/2
  Demux/2 -> Moment/1  "Moment"
  Add/1 -> Demux/1
  Demux1/2 -> Mux1/2
  Product/1 -> Sum/1  "Gravity_Force"
  Thrust_Force&Moment/1 -> Add/2
  Sum/1 -> Force/1  "Force"
  Demux/1 -> Divide/1, Sum/2
  Gain1/1 -> Mux1/3
  Demux1/1 -> Mux1/1
  Gain/1 -> Mux/3, Divide/2  "weight"
  Aero_Force&Moment/1 -> Add/1
  mass/1 -> Gain/1
  Constant/1 -> Mux/1, Mux/2
  Divide/1 -> Demux1/1
  R_EB/1 -> Product/1

== system f18_SimulationModel/f18 Model/6DoF_Model/Subsystem3 ==
  VelocityInertial : Inport
  Add : Sum
  Atan1 : Trigonometry  Operator=atan2
  Atan2 : Trigonometry  Operator=atan2
  Demux : Demux  Outputs=3
  Gain1 : Gain  Gain=180/pi
  Gain2 : Gain  Gain=180/pi
  Sqrt : Sqrt
  Square : Math  Operator=square
  Square1 : Math  Operator=square
  GroundSpeed : Outport
  ClimbAngle : Outport  Port=2
  TrackAngle : Outport  Port=3
  wires:
  VelocityInertial/1 -> Demux/1
  Atan1/1 -> Gain2/1
  Square/1 -> Add/1
  Demux/3 -> Atan2/1  "Zdot_E"
  Add/1 -> Sqrt/1
  Atan2/1 -> Gain1/1
  Square1/1 -> Add/2
  Sqrt/1 -> Atan2/2, GroundSpeed/1
  Demux/1 -> Square/1, Atan1/2  "Xdot_E"
  Demux/2 -> Square1/1, Atan1/1  "Ydot_E"
  Gain1/1 -> ClimbAngle/1
  Gain2/1 -> TrackAngle/1

== system f18_SimulationModel/f18 Model/Aerodynamic_Model/Absolute Force&Moment ==
  rhoh : Inport
  TAS : Inport  Port=2
  CF : Inport  Port=3
  CM : Inport  Port=4
  Constant : Constant  Value=b
  Constant1 : Constant  Value=cbar
  Demux1 : Demux  Outputs=3
  Demux2 : Demux  Outputs=3
  Mux : Mux  Inputs=6
  Product : Product
  Product1 : Product  Inputs=3
  Product2 : Product  Inputs=3
  Product3 : Product  Inputs=3
  Subsystem1 : Subsystem
  Aero_Force&Moment_ac : Outport
  wires:
  Demux2/3 -> Product3/2
  Demux1/3 -> Mux/3  "Z_aero"
  Constant1/1 -> Product2/3
  CF/1 -> Product/2
  CM/1 -> Demux2/1
  Demux1/1 -> Mux/1  "X_aero"
  Product3/1 -> Mux/6  "N_aero"
  Subsystem1/1(QS) -> [QS]  "QS"
  Constant/1 -> Product3/3, Product1/3
  Product/1 -> Demux1/1  "Aero_Forces"
  Demux2/1 -> Product1/2  "Cl"
  Demux2/2 -> Product2/2
  [QS] -> Product3/1, Product2/1, Product1/1
  Product2/1 -> Mux/5  "M_aero"
  Demux1/2 -> Mux/2  "Y_aero"
  Product1/1 -> Mux/4  "L_aero"
  rhoh/1 -> Subsystem1/1(rhoh)
  [QS] -> Product/1
  TAS/1 -> Subsystem1/2(TAS)
  Mux/1 -> Aero_Force&Moment_ac/1  "Aero_Force&Moment_ac"

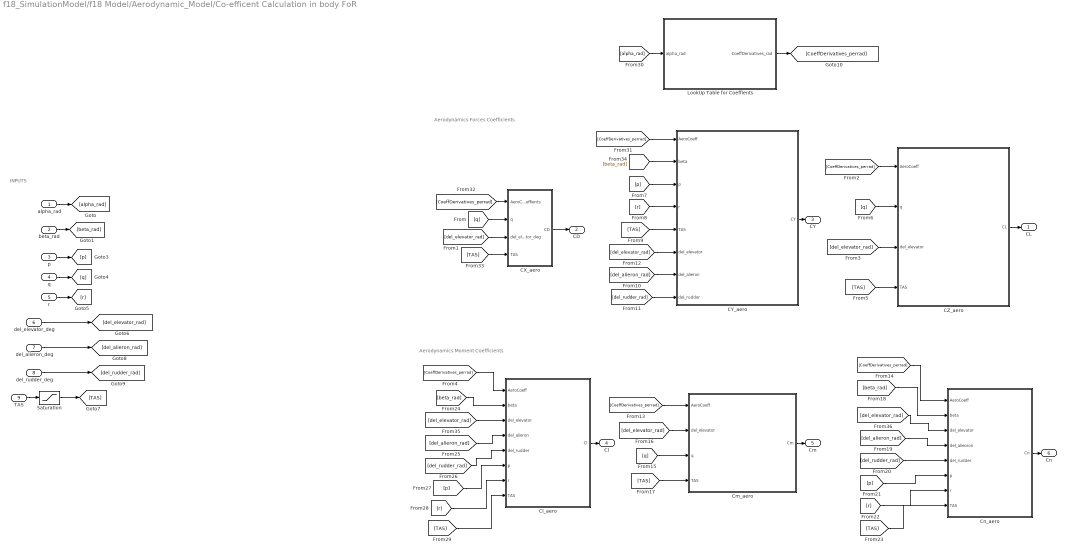
== system f18_SimulationModel/f18 Model/Aerodynamic_Model/Co-efficent Calculation in body FoR ==
  note: INPUTS
  note: Aerodynamics Moment Coefficients
  note: Aerodynamics Forces Coefficients
  alpha_rad : Inport
  beta_rad : Inport  Port=2
  p : Inport  Port=3
  q : Inport  Port=4
  r : Inport  Port=5
  del_elevator_deg : Inport  Port=6
  del_alieron_deg : Inport  Port=7
  del_rudder_deg : Inport  Port=8
  TAS : Inport  Port=9
  CX_aero : Subsystem
  CY_aero : Subsystem
  CZ_aero : Subsystem
  Cl_aero : Subsystem
  Cm_aero : Subsystem
  Cn_aero : Subsystem
  LookUp Table for Coeffients : Subsystem
  Saturation : Saturate  UpperLimit=inf  LowerLimit=0.1
  CL : Outport
  CD : Outport  Port=2
  CY : Outport  Port=3
  Cl : Outport  Port=4
  Cm : Outport  Port=5
  Cn : Outport  Port=6
  wires:
  Saturation/1 -> [TAS]
  [del_elevator_rad] -> CZ_aero/3(del_elevator)
  alpha_rad/1 -> [alpha_rad]
  TAS/1 -> Saturation/1
  [r] -> Cn_aero/7(r)
  q/1 -> [q]
  beta_rad/1 -> [beta_rad]
  [r] -> Cl_aero/7(r)
  p/1 -> [p]
  [q] -> Cm_aero/3(q)
  [del_elevator_rad] -> CX_aero/3(del_elevator_deg)
  [del_elevator_rad] -> Cm_aero/2(del_elevator)
  Cm_aero/1(Cm) -> Cm/1
  [del_rudder_rad] -> Cl_aero/5(del_rudder)
  [TAS] -> Cm_aero/4(TAS)
  [TAS] -> Cl_aero/8(TAS)
  [beta_rad] -> Cl_aero/2(beta)
  [del_rudder_rad] -> Cn_aero/5(del_rudder)
  [p] -> Cl_aero/6(p)
  [beta_rad] -> Cn_aero/2(beta)
  [del_alieron_rad] -> Cl_aero/4(del_alieron)
  r/1 -> [r]
  [TAS] -> CZ_aero/4(TAS)
  Cl_aero/1(Cl) -> Cl/1
  [del_alieron_rad] -> Cn_aero/4(del_alieoron)
  [p] -> Cn_aero/6(p)
  [TAS] -> Cn_aero/8(TAS)
  [q] -> CZ_aero/2(q)
  Cn_aero/1(Cn) -> Cn/1
  CX_aero/1(CD) -> CD/1
  CY_aero/1(CY) -> CY/1
  CZ_aero/1(CL) -> CL/1
  [alpha_rad] -> LookUp Table for Coeffients/1(alpha_rad)
  LookUp Table for Coeffients/1(CoeffDerivatives_rad) -> [CoeffDerivatives_perrad]
  [CoeffDerivatives_perrad] -> CX_aero/1(AeroCoeffients)
  [TAS] -> CX_aero/4(TAS)
  [q] -> CX_aero/2(q)
  [CoeffDerivatives_perrad] -> CY_aero/1(AeroCoeff)
  [p] -> CY_aero/3(p)
  [r] -> CY_aero/4(r)
  [TAS] -> CY_aero/5(TAS)
  [del_alieron_rad] -> CY_aero/7(del_alieron)
  [del_rudder_rad] -> CY_aero/8(del_rudder)
  [del_elevator_rad] -> CY_aero/6(del_elevator)
  [beta_rad] -> CY_aero/2(beta)
  [CoeffDerivatives_perrad] -> CZ_aero/1(AeroCoeff)
  [CoeffDerivatives_perrad] -> Cl_aero/1(AeroCoeff)
  [CoeffDerivatives_perrad] -> Cm_aero/1(AeroCoeff)
  [CoeffDerivatives_perrad] -> Cn_aero/1(AeroCoeff)
  [del_elevator_rad] -> Cl_aero/3(del_elevator)
  [del_elevator_rad] -> Cn_aero/3(del_elevator)
  del_elevator_deg/1 -> [del_elevator_rad]
  del_alieron_deg/1 -> [del_alieron_rad]
  del_rudder_deg/1 -> [del_rudder_rad]

== system f18_SimulationModel/f18 Model/Aerodynamic_Model/Stability FoR to Body FoR ==
  note: Cx = -CD
      | Cz = -CL
  note: In stability FoR
      | at AC
  note: In body FoR
      | at AC
  alpha_rad : Inport
  CL : Inport  Port=2
  CD : Inport  Port=3
  CY : Inport  Port=4
  Cl : Inport  Port=5
  Cm : Inport  Port=6
  Cn : Inport  Port=7
  Demux : Demux  Outputs=3
  Gain : Gain  Gain=-1
  Gain1 : Gain  Gain=-1
  Matrix Multiply : Product  Multiplication=Matrix(*)
  Matrix Multiply1 : Product  Multiplication=Matrix(*)
  Mux : Mux  Inputs=3
  Mux1 : Mux  Inputs=3
  Mux2 : Mux  Inputs=3
  StabilityToBody : Rotation_Matrices_All/StabilityToBody  SystemSampleTime=-1  VariantActivationTime=update diagram  AllowFlexibleInterface=on  Latency=0  AutoFrameSizeCalculation=off
  AeroForce_Coefficients_bFoR : Outport
  AeroMoment_Coefficients_b_AC : Outport  Port=2
  wires:
  Mux/1 -> Matrix Multiply/2  "AeroForce_Coefficients_sFoR"
  Cm/1 -> Mux1/2
  Mux1/1 -> Matrix Multiply1/2  "AeroMoment_Coefficients_sFoR"
  alpha_rad/1 -> StabilityToBody/1
  Cn/1 -> Mux1/3
  Cl/1 -> Mux1/1
  Matrix Multiply1/1 -> AeroMoment_Coefficients_b_AC/1  "AeroMoment_Coefficients_b_AC"
  CD/1 -> Mux/1
  CY/1 -> Mux/2
  CL/1 -> Mux/3
  Matrix Multiply/1 -> Demux/1
  Demux/1 -> Gain/1
  Mux2/1 -> AeroForce_Coefficients_bFoR/1  "AeroForce_Coefficients_bFoR"
  Gain/1 -> Mux2/1
  Demux/2 -> Mux2/2
  Demux/3 -> Gain1/1
  Gain1/1 -> Mux2/3
  StabilityToBody/1 -> Matrix Multiply1/1, Matrix Multiply/1

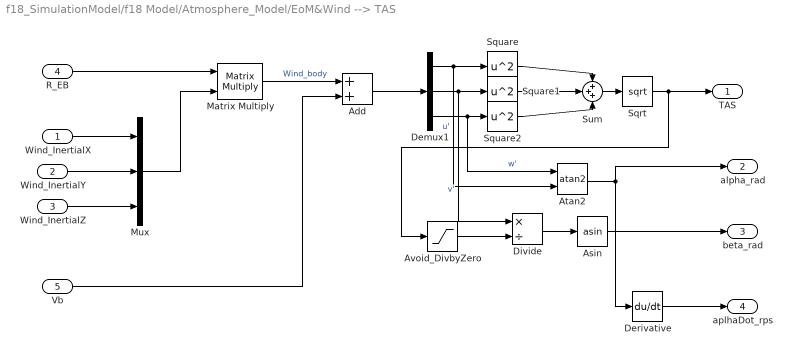
== system f18_SimulationModel/f18 Model/Atmosphere_Model/EoM&Wind --> TAS ==
  Wind_InertialX : Inport
  Wind_InertialY : Inport  Port=2
  Wind_InertialZ : Inport  Port=3
  R_EB : Inport  Port=4
  Vb : Inport  Port=5
  Add : Sum
  Asin : Trigonometry  Operator=asin
  Atan2 : Trigonometry  Operator=atan2
  Avoid_DivbyZero : Saturate  UpperLimit=inf  LowerLimit=0.1
  Demux1 : Demux  Outputs=3
  Derivative : Derivative
  Divide : Product  Inputs=*/
  Matrix Multiply : Product  Multiplication=Matrix(*)
  Mux : Mux  Inputs=3
  Sqrt : Sqrt
  Square : Math  Operator=square
  Square1 : Math  Operator=square
  Square2 : Math  Operator=square
  Sum : Sum  Inputs=+++
  TAS : Outport
  alpha_rad : Outport  Port=2
  beta_rad : Outport  Port=3
  aplhaDot_rps : Outport  Port=4
  wires:
  Avoid_DivbyZero/1 -> Divide/2
  Divide/1 -> Asin/1
  Sum/1 -> Sqrt/1
  Wind_InertialX/1 -> Mux/1
  Demux1/1 -> Atan2/2, Square/1  "u'"
  Demux1/3 -> Atan2/1, Square2/1  "w'"
  Matrix Multiply/1 -> Add/1  "Wind_body"
  Atan2/1 -> alpha_rad/1, Derivative/1
  Sqrt/1 -> TAS/1, Avoid_DivbyZero/1
  Square/1 -> Sum/1
  Mux/1 -> Matrix Multiply/2
  Demux1/2 -> Divide/1, Square1/1  "v'"
  Square1/1 -> Sum/2
  Derivative/1 -> aplhaDot_rps/1
  Wind_InertialY/1 -> Mux/2
  Vb/1 -> Add/2
  Add/1 -> Demux1/1
  Asin/1 -> beta_rad/1
  R_EB/1 -> Matrix Multiply/1
  Wind_InertialZ/1 -> Mux/3
  Square2/1 -> Sum/3

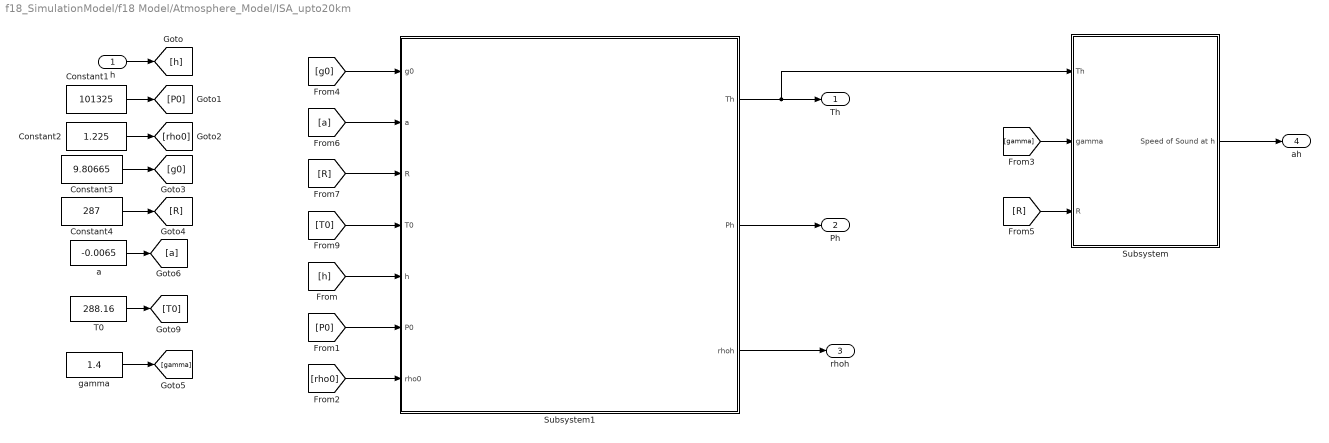
== system f18_SimulationModel/f18 Model/Atmosphere_Model/ISA_upto20km ==
  h : Inport
  Constant1 : Constant  Value=101325
  Constant2 : Constant  Value=1.225
  Constant3 : Constant  Value=9.80665
  Constant4 : Constant  Value=287
  Subsystem : Subsystem
  Subsystem1 : Subsystem
  T0 : Constant  Value=288.16
  a : Constant  Value=-0.0065
  gamma : Constant  Value=1.4
  Th : Outport
  Ph : Outport  Port=2
  rhoh : Outport  Port=3
  ah : Outport  Port=4
  wires:
  gamma/1 -> [gamma]
  a/1 -> [a]
  Constant1/1 -> [P0]
  Constant4/1 -> [R]
  Constant2/1 -> [rho0]
  Constant3/1 -> [g0]
  h/1 -> [h]
  T0/1 -> [T0]
  [g0] -> Subsystem1/1(g0)
  [a] -> Subsystem1/2(a)
  [R] -> Subsystem1/3(R)
  [T0] -> Subsystem1/4(T0)
  [h] -> Subsystem1/5(h)
  [P0] -> Subsystem1/6(P0)
  [rho0] -> Subsystem1/7(rho0)
  Subsystem1/1(Th) -> Subsystem/1(Th), Th/1
  Subsystem1/2(Ph) -> Ph/1
  Subsystem1/3(rhoh) -> rhoh/1
  Subsystem/1(Speed of Sound at h) -> ah/1
  [gamma] -> Subsystem/2(gamma)
  [R] -> Subsystem/3(R)

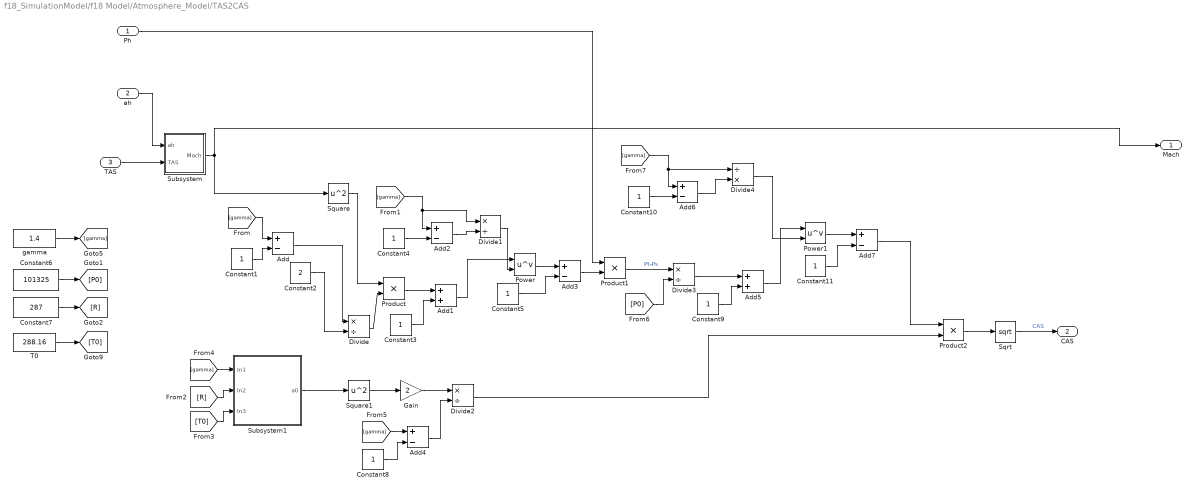
== system f18_SimulationModel/f18 Model/Atmosphere_Model/TAS2CAS ==
  Ph : Inport
  ah : Inport  Port=2
  TAS : Inport  Port=3
  Add{,2..4,6..7} (6 alike) : Sum  Inputs=+-
  Add1 : Sum
  Add5 : Sum
  Constant{1,3..5,8..11} (8 alike) : Constant
  Constant2 : Constant  Value=2
  Constant6 : Constant  Value=101325
  Constant7 : Constant  Value=287
  Divide{,1..3} (4 alike) : Product  Inputs=*/
  Divide4 : Product  Inputs=/*
  Gain : Gain  Gain=2
  Power : Math  Operator=pow
  Power1 : Math  Operator=pow
  Product : Product
  Product1 : Product
  Product2 : Product
  Sqrt : Sqrt
  Square : Math  Operator=square
  Square1 : Math  Operator=square
  Subsystem : Subsystem
  Subsystem1 : Subsystem
  T0 : Constant  Value=288.16
  gamma : Constant  Value=1.4
  Mach : Outport
  CAS : Outport  Port=2
  wires:
  [gamma] -> Add6/1, Divide4/1
  [P0] -> Divide3/2
  Square1/1 -> Gain/1
  Product/1 -> Add1/1
  Constant3/1 -> Add1/2
  Add1/1 -> Power/1
  Constant2/1 -> Divide/2
  gamma/1 -> [gamma]
  Constant11/1 -> Add7/2
  Add/1 -> Divide/1
  Gain/1 -> Divide2/1
  Constant8/1 -> Add4/2
  Subsystem/1(Mach) -> Mach/1, Square/1
  Constant7/1 -> [R]
  [gamma] -> Add2/1, Divide1/1
  Constant6/1 -> [P0]
  Constant9/1 -> Add5/2
  Add7/1 -> Product2/1
  Divide4/1 -> Power1/2
  Add3/1 -> Product1/2
  Constant5/1 -> Add3/2
  Add4/1 -> Divide2/2
  Add2/1 -> Divide1/2
  Add5/1 -> Power1/1
  [gamma] -> Add/1
  Divide1/1 -> Power/2
  Divide3/1 -> Add5/1
  Subsystem1/1(a0) -> Square1/1
  Power1/1 -> Add7/1
  Constant1/1 -> Add/2
  Ph/1 -> Product1/1
  [gamma] -> Add4/1
  T0/1 -> [T0]
  [T0] -> Subsystem1/3(In3)
  Product1/1 -> Divide3/1  "Pt-Ps"
  TAS/1 -> Subsystem/2(TAS)
  [gamma] -> Subsystem1/1(In1)
  [R] -> Subsystem1/2(In2)
  Constant10/1 -> Add6/2
  Sqrt/1 -> CAS/1  "CAS"
  Add6/1 -> Divide4/2
  Power/1 -> Add3/1
  ah/1 -> Subsystem/1(ah)
  Divide/1 -> Product/2
  Constant4/1 -> Add2/2
  Square/1 -> Product/1
  Product2/1 -> Sqrt/1
  Divide2/1 -> Product2/2

== system f18_SimulationModel/f18 Model/6DoF_Model/6DoF_EoM/Rotational_EoM ==
  Moment : Inport
  Inertia : Inport  Port=2
  Add : Sum  Inputs=+-
  Cross Product : matrix_library/Cross Product
  Demux : Demux  Outputs=3
  Divide : Product  Inputs=/*  Multiplication=Matrix(*)
  Mux : Mux  Inputs=3
  Product : Product  Multiplication=Matrix(*)
  p_dot : Integrator  InitialCondition=init_omega_b(1)  ContinuousStateAttributes='p_dot'
  q_dot : Integrator  InitialCondition=init_omega_b(2)  ContinuousStateAttributes='q_dot'
  r_dot : Integrator  InitialCondition=init_omega_b(3)  ContinuousStateAttributes='r_dot'
  omega_b : Outport
  wires:
  Moment/1 -> Add/1
  Product/1 -> Cross Product/2
  q_dot/1 -> Mux/2  "q"
  Divide/1 -> Demux/1
  Demux/1 -> p_dot/1  "p_dot"
  Cross Product/1 -> Add/2
  Inertia/1 -> Divide/1, Product/1
  r_dot/1 -> Mux/3  "r"
  Demux/2 -> q_dot/1  "q_dot"
  Demux/3 -> r_dot/1  "r_dot"
  Mux/1 -> Product/2, Cross Product/1, omega_b/1  "omega_b"
  p_dot/1 -> Mux/1  "p"
  Add/1 -> Divide/2

== system f18_SimulationModel/f18 Model/6DoF_Model/6DoF_EoM/Translational_EoM ==
  Force : Inport
  omega : Inport  Port=2
  Add : Sum  Inputs=+-
  Constant : Constant  Value=mass
  Cross Product : matrix_library/Cross Product
  Demux : Demux  Outputs=3
  Divide : Product  Inputs=*/
  Mux1 : Mux  Inputs=3
  u_dot : Integrator  InitialCondition=init_Vb(1)  ContinuousStateAttributes='u_dot'
  v_dot : Integrator  InitialCondition=init_Vb(2)  ContinuousStateAttributes='v_dot'
  w_dot : Integrator  InitialCondition=init_Vb(3)  ContinuousStateAttributes='w_dot'
  V_b : Outport
  wires:
  omega/1 -> Cross Product/1  "omega"
  Demux/1 -> u_dot/1  "u_dot"
  Demux/3 -> w_dot/1  "w_dot"
  Cross Product/1 -> Add/2
  w_dot/1 -> Mux1/3  "w"
  Demux/2 -> v_dot/1  "v_dot"
  Mux1/1 -> Cross Product/2, V_b/1  "V_b"
  u_dot/1 -> Mux1/1  "u"
  Add/1 -> Demux/1
  v_dot/1 -> Mux1/2  "v"
  Force/1 -> Divide/1  "Force"
  Divide/1 -> Add/1
  Constant/1 -> Divide/2

== system f18_SimulationModel/f18 Model/6DoF_Model/EarthToBody/Subsystem2 ==
  note: Reshape creates array by arranging them in column first manner
  psi : Inport
  Constant{10..11,13..14} (4 alike) : Constant  Value=0
  Constant12 : Constant
  Cos : Trigonometry  Operator=cos
  Gain1 : Gain  Gain=-1
  Mux2 : Mux  Inputs=9
  Reshape2 : Reshape  OutputDimensionality=Customize  OutputDimensions=[3,3]
  Sin : Trigonometry
  Transpose : Math  Operator=transpose
  R_psi : Outport
  wires:
  Transpose/1 -> R_psi/1
  [cosPSI] -> Mux2/5
  Gain1/1 -> Mux2/4
  Constant11/1 -> Mux2/7
  Constant14/1 -> Mux2/8
  Constant12/1 -> Mux2/9
  Constant13/1 -> Mux2/6
  Mux2/1 -> Reshape2/1
  Reshape2/1 -> Transpose/1
  Sin/1 -> [sinPSI]
  Cos/1 -> [cosPSI]
  Constant10/1 -> Mux2/3
  [cosPSI] -> Mux2/1
  [sinPSI] -> Gain1/1
  [sinPSI] -> Mux2/2
  psi/1 -> Cos/1, Sin/1

== system f18_SimulationModel/f18 Model/6DoF_Model/EarthToBody/Subsystem3 ==
  note: Reshape creates array by arranging them in column first manner
  phi : Inport
  Constant1 : Constant
  Constant{2..3,10..11} (4 alike) : Constant  Value=0
  Cos2 : Trigonometry  Operator=cos
  Gain2 : Gain  Gain=-1
  Mux2 : Mux  Inputs=9
  Reshape2 : Reshape  OutputDimensionality=Customize  OutputDimensions=[3,3]
  Sin2 : Trigonometry
  Transpose : Math  Operator=transpose
  R_phi : Outport
  wires:
  Gain2/1 -> Mux2/8
  Cos2/1 -> [cosPHI]
  Sin2/1 -> [sinPHI]
  phi/1 -> Cos2/1, Sin2/1
  Constant2/1 -> Mux2/2
  Constant1/1 -> Mux2/1
  Constant10/1 -> Mux2/3
  Reshape2/1 -> Transpose/1
  Mux2/1 -> Reshape2/1
  [sinPHI] -> Mux2/6
  [cosPHI] -> Mux2/9
  [sinPHI] -> Gain2/1
  Constant11/1 -> Mux2/7
  Constant3/1 -> Mux2/4
  [cosPHI] -> Mux2/5
  Transpose/1 -> R_phi/1

== system f18_SimulationModel/f18 Model/6DoF_Model/EarthToBody/Subsystem4 ==
  note: Reshape creates array by arranging them in column first manner
  theta : Inport
  Constant{1..3,5} (4 alike) : Constant  Value=0
  Constant4 : Constant
  Cos1 : Trigonometry  Operator=cos
  Gain1 : Gain  Gain=-1
  Mux2 : Mux  Inputs=9
  Reshape2 : Reshape  OutputDimensionality=Customize  OutputDimensions=[3,3]
  Sin1 : Trigonometry
  Transpose : Math  Operator=transpose
  R_theta : Outport
  wires:
  Gain1/1 -> Mux2/3
  Cos1/1 -> [cosTHETA]
  theta/1 -> Cos1/1, Sin1/1
  Sin1/1 -> [sinTHETA]
  Transpose/1 -> R_theta/1
  Constant4/1 -> Mux2/5
  Constant3/1 -> Mux2/4
  [sinTHETA] -> Mux2/7
  [cosTHETA] -> Mux2/9
  Constant1/1 -> Mux2/6
  Mux2/1 -> Reshape2/1
  Reshape2/1 -> Transpose/1
  [sinTHETA] -> Gain1/1
  [cosTHETA] -> Mux2/1
  Constant2/1 -> Mux2/2
  Constant5/1 -> Mux2/8

== system f18_SimulationModel/f18 Model/Aerodynamic_Model/Absolute Force&Moment/Subsystem1 ==
  rhoh : Inport
  TAS : Inport  Port=2
  Gain : Gain  Gain=1/2
  Product : Product
  Product1 : Product
  Square : Math  Operator=square
  WingArea : Constant  Value=S
  QS : Outport
  wires:
  TAS/1 -> Square/1
  Product/1 -> Product1/2  "Q"
  rhoh/1 -> Gain/1
  Gain/1 -> Product/1
  WingArea/1 -> Product1/1
  Product1/1 -> QS/1  "QS"
  Square/1 -> Product/2

== system f18_SimulationModel/f18 Model/Aerodynamic_Model/Co-efficent Calculation in body FoR/CX_aero ==
  AeroCoeffients : Inport
  q : Inport  Port=2
  del_elevator_deg : Inport  Port=3
  TAS : Inport  Port=4
  Add : Sum  Inputs=+++
  Bus Selector : BusSelector  OutputSignals=CD0,CD_q,CD_de
  Divide : Product  Inputs=*/
  Gain : Gain  Gain=cbar/2
  Product1 : Product
  Product2 : Product
  CD : Outport
  wires:
  Add/1 -> CD/1  "CD"
  AeroCoeffients/1 -> Bus Selector/1
  Bus Selector/1 -> Add/1  "<CD0>"
  TAS/1 -> Divide/2
  q/1 -> Gain/1
  Product1/1 -> Divide/1
  Bus Selector/2 -> Product1/1  "<CD_q>"
  Gain/1 -> Product1/2
  Divide/1 -> Add/2
  del_elevator_deg/1 -> Product2/2
  Bus Selector/3 -> Product2/1  "<CD_de>"
  Product2/1 -> Add/3
